simulink model "soc_WLAN_fpga"  (R2024b)
settings: Solver=FixedStepDiscrete  StartTime=0.0  StopTime=stopTime  RelTol=1e-3
PreLoadFcn:
  | addpath(fullfile(matlabroot,'toolbox','whdl','whdlexamples','whdlexamples'));
InitFcn:
  | addpath(fullfile(matlabroot,'toolbox','whdl','whdlexamples','whdlexamples'));
model workspace (MAT data in the model file):
  socvcb : containers.Map (value not decoded)
undefined symbols (not defined in the file): Add, bitRatePerOfdmSym, chanBW, coe, cpLen, dataUpsampleFactor, DelayValMaxNsdMinusLastPilotSc, DescramblerInitialSeed, designMultirateFIR, fftLen, filterLatency, filterUpsampleFactor, Fs, Hd, HT_MFMCS0, HT_MFMCS1, HT_MFMCS2, HT_MFMCS3, HT_MFMCS4, HT_MFMCS5, HT_MFMCS6, HT_MFMCS7, HTUnUsedScInd, inputSamplingRate, interp_coeff, maxPilotRefCounterVale, maxPilotsRef, maxPilotsRefNonHT, Ncol_HT, Ncol_NonHT, noDataSubCarriers, Non_HTMCS0, Non_HTMCS1, Non_HTMCS2, Non_HTMCS3, Non_HTMCS4, Non_HTMCS5, Non_HTMCS6, Non_HTMCS7, Nrow_HT, Nrow_NonHT, numDSC_HT, numDSC_HT_vhtSigB, numDSC_NonHT, numDscHT, numDscNonHT, numOfBitsPerOFDMSym, numOfDataBitsPerOFDMSym, numPilots, numScHT, numSCS_HT, numSCS_NonHT, pnSeq, QAM, rxDownsampleFactor, secondPIdx_HT, secondPIdx_NonHT, Shift, VHTMCS0, VHTMCS1 ... (+7)
libraries: hdlsllib x267, simulink x210, dspsigops x22, whdlutilities x10, whdlmod x9, dsphdlfiltering2 x5, dsphdlmathfun2 x4, whdledac x3, hwlogicconnlib x2, commhdlcrc x2, dsphdlsigops2 x2
(part 10 of 14)

== system soc_WLAN_fpga/WLAN/WLAN HDL/WLAN_Tx_Rx/WLAN_Rx/WLANHDLReceiver/DataRecovery/Deinterleaver/DeInterleaver_HT/Stage 2 64QAM/Write Logic/Handle Input Control Signals ==
  start : Inport
  valid : Inport  Port=2
  end : Inport  Port=3
  Delay{1..5} (5 alike) : Delay  DelayLength=1
  Generate Current Frame Status : Subsystem
  Generate Forced End : Subsystem
  Logical Operator : Logic  Operator=OR  IconShape=distinctive  AllPortsSameDT=off  OutDataTypeStr=boolean
  Logical Operator1 : Logic  Operator=NOT  IconShape=distinctive  AllPortsSameDT=off  OutDataTypeStr=boolean
  Logical Operator2 : Logic  IconShape=distinctive  AllPortsSameDT=off  OutDataTypeStr=boolean
  Logical Operator3 : Logic  Inputs=4  IconShape=distinctive  AllPortsSameDT=off  OutDataTypeStr=boolean
  Logical Operator5 : Logic  IconShape=distinctive  AllPortsSameDT=off  OutDataTypeStr=boolean
  reset : Outport
  countEnb : Outport  Port=2
  endOut : Outport  Port=3
  endReady : Outport  Port=4
  wires:
  Logical Operator1/1 -> Logical Operator3/4
  Logical Operator/1 -> Delay1/1, endReady/1
  Delay1/1 -> Generate Current Frame Status/2(end), Delay5/1, Logical Operator1/1
  Generate Forced End/1(forcedEnd) -> Logical Operator/2
  Logical Operator3/1 -> Logical Operator/1
  valid/1 -> Logical Operator3/1, Logical Operator2/2, Generate Forced End/2(valid), Delay4/1
  Delay5/1 -> endOut/1
  Delay3/1 -> countEnb/1
  Delay2/1 -> reset/1
  start/1 -> Logical Operator2/1
  Delay4/1 -> Logical Operator5/1
  end/1 -> Logical Operator3/2
  Logical Operator2/1 -> Generate Forced End/1(rst), Generate Current Frame Status/1(start), Delay2/1
  Generate Current Frame Status/1(frameOn) -> Generate Forced End/3(frameOn), Logical Operator3/3, Logical Operator5/2
  Logical Operator5/1 -> Delay3/1

== system soc_WLAN_fpga/WLAN/WLAN HDL/WLAN_Tx_Rx/WLAN_Rx/WLANHDLReceiver/DataRecovery/Deinterleaver/DeInterleaver_HT/Stage 2 BPSK/Generate Ready/Generate Ready2 ==
  fifoCount : Inport
  pop : Inport  Port=2
  Compare To Constant1 : simulink/Logic and Bit Operations/Compare To Constant  relop===  const=0  OutDataTypeStr=boolean
  Compare To Constant4 : simulink/Logic and Bit Operations/Compare To Constant  relop===  const=1  OutDataTypeStr=boolean
  Logical Operator1 : Logic  Operator=OR  IconShape=distinctive  AllPortsSameDT=off  OutDataTypeStr=boolean
  Logical Operator14 : Logic  IconShape=distinctive  AllPortsSameDT=off  OutDataTypeStr=boolean
  ready2 : Outport
  wires:
  Compare To Constant1/1 -> Logical Operator1/1
  Logical Operator1/1 -> ready2/1
  Logical Operator14/1 -> Logical Operator1/2
  Compare To Constant4/1 -> Logical Operator14/1
  pop/1 -> Logical Operator14/2
  fifoCount/1 -> Compare To Constant4/1, Compare To Constant1/1

== system soc_WLAN_fpga/WLAN/WLAN HDL/WLAN_Tx_Rx/WLAN_Rx/WLANHDLReceiver/DataRecovery/Deinterleaver/DeInterleaver_HT/Stage 2 BPSK/Read Logic/Generate Base Read Address ==
  readStart : Inport
  Constant1 : Constant  Value=0  OutDataTypeStr=fixdt(0,nextpow2(maxBlkSize+1),0)  SampleTime=-1
  Constant5 : Constant  Value=maxBlkSize  OutDataTypeStr=fixdt(0,nextpow2(maxBlkSize+1),0)  SampleTime=-1
  Logical Operator7 : Logic  Operator=NOT  IconShape=distinctive  AllPortsSameDT=off  OutDataTypeStr=boolean
  Switch1 : Switch  Criteria=u2 ~= 0  SaturateOnIntegerOverflow=off  InputSameDT=off
  Unit Delay Enabled Synchronous2 : hdlsllib/Discrete/Unit Delay Enabled Synchronous  InitialCondition=1  SampleTime=-1
  baseAddr : Outport
  wires:
  readStart/1 -> Unit Delay Enabled Synchronous2/2
  Logical Operator7/1 -> Unit Delay Enabled Synchronous2/1
  Switch1/1 -> baseAddr/1
  Constant5/1 -> Switch1/1
  Constant1/1 -> Switch1/3
  Unit Delay Enabled Synchronous2/1 -> Logical Operator7/1, Switch1/2

== system soc_WLAN_fpga/WLAN/WLAN HDL/WLAN_Tx_Rx/WLAN_Rx/WLANHDLReceiver/DataRecovery/Deinterleaver/DeInterleaver_HT/Stage 2 BPSK/Read Logic/Generate Output Control Signals ==
  blockLen : Inport
  blockValid : Inport  Port=2
  blockCount : Inport  Port=3
  Add : Sum  Inputs=+-
  Add1 : Sum  Inputs=+-
  Compare To Constant : simulink/Logic and Bit Operations/Compare To Constant  relop===  const=0  OutDataTypeStr=boolean
  Constant : Constant  Value=8  OutDataTypeStr=fixdt(0,nextpow2(8+1),0)  SampleTime=-1
  Constant1 : Constant  Value=false  SampleTime=-1
  Constant2 : Constant  Value=11  OutDataTypeStr=fixdt(0,nextpow2(11+1),0)  SampleTime=-1
  Constant3 : Constant  Value=false  SampleTime=-1
  Delay{,1,5..6,8} (5 alike) : Delay  DelayLength=1
  Logical Operator1 : Logic  IconShape=distinctive  AllPortsSameDT=off  OutDataTypeStr=boolean
  Logical Operator2 : Logic  IconShape=distinctive  AllPortsSameDT=off  OutDataTypeStr=boolean
  Logical Operator3 : Logic  Operator=NOR  IconShape=distinctive  AllPortsSameDT=off  OutDataTypeStr=boolean
  Logical Operator4 : Logic  Operator=OR  IconShape=distinctive  AllPortsSameDT=off  OutDataTypeStr=boolean
  Logical Operator8 : Logic  IconShape=distinctive  AllPortsSameDT=off  OutDataTypeStr=boolean
  Relational Operator : RelationalOperator  Operator===  OutDataTypeStr=boolean  InputSameDT=off
  Relational Operator1 : RelationalOperator  OutDataTypeStr=boolean  InputSameDT=off
  Relational Operator2 : RelationalOperator  Operator=<=  OutDataTypeStr=boolean  InputSameDT=off
  Relational Operator3 : RelationalOperator  OutDataTypeStr=boolean  InputSameDT=off
  Unit Delay Enabled Synchronous : hdlsllib/Discrete/Unit Delay Enabled Synchronous  InitialCondition=1  SampleTime=-1
  Unit Delay Enabled Synchronous1 : hdlsllib/Discrete/Unit Delay Enabled Synchronous  InitialCondition=1  SampleTime=-1
  start : Outport
  end : Outport  Port=2
  valid : Outport  Port=3
  pop : Outport  Port=4
  advPop : Outport  Port=5
  wires:
  blockLen/1 -> Relational Operator/2, Add/1, Add1/1, Relational Operator2/2
  Delay/1 -> start/1, Unit Delay Enabled Synchronous/2, Unit Delay Enabled Synchronous1/2
  blockCount/1 -> Compare To Constant/1, Relational Operator/1, Relational Operator2/1, Relational Operator1/1, Relational Operator3/1
  Unit Delay Enabled Synchronous1/1 -> Logical Operator3/2
  Relational Operator3/1 -> Delay1/1
  Add1/1 -> Relational Operator3/2
  Constant2/1 -> Add1/2
  Constant3/1 -> Unit Delay Enabled Synchronous1/1
  Delay1/1 -> Logical Operator3/1
  Logical Operator3/1 -> advPop/1
  Unit Delay Enabled Synchronous/1 -> Logical Operator4/2
  Delay8/1 -> Logical Operator4/1
  Logical Operator4/1 -> pop/1
  Delay6/1 -> valid/1
  Delay5/1 -> end/1
  Constant1/1 -> Unit Delay Enabled Synchronous/1
  Compare To Constant/1 -> Logical Operator8/2
  Relational Operator1/1 -> Delay8/1
  Add/1 -> Relational Operator1/2
  Constant/1 -> Add/2
  Relational Operator2/1 -> Logical Operator1/2
  Relational Operator/1 -> Logical Operator2/2
  blockValid/1 -> Logical Operator8/1, Logical Operator2/1, Logical Operator1/1
  Logical Operator2/1 -> Delay5/1
  Logical Operator8/1 -> Delay/1
  Logical Operator1/1 -> Delay6/1

== system soc_WLAN_fpga/WLAN/WLAN HDL/WLAN_Tx_Rx/WLAN_Rx/WLANHDLReceiver/DataRecovery/Deinterleaver/DeInterleaver_HT/Stage 2 BPSK/Read Logic/Generate Read Address ==
  note: 1) Add Subsystem or Model blocks as valid variant choices.
      | 2) You cannot connect blocks at this level. At simulation, connectivity is automatically
      | determined, based on the active variant and port name matching.
  blockLen : Inport
  enable : Inport  Port=2
  reset : Inport  Port=3
  Read Address of Deinterleaver : Subsystem  VariantControl=isInterleaver==0
  Read Address of Interleaver : Subsystem  VariantControl=isInterleaver==1
  blockDataCount : Outport
  currentAddr : Outport  Port=2

== system soc_WLAN_fpga/WLAN/WLAN HDL/WLAN_Tx_Rx/WLAN_Rx/WLANHDLReceiver/DataRecovery/Deinterleaver/DeInterleaver_HT/Stage 2 BPSK/Write Logic/Generate Write Address ==
  rst : Inport
  enb : Inport  Port=2
  end : Inport  Port=3
  Add : Sum  OutDataTypeStr=Inherit: Inherit via back propagation
  Constant : Constant  Value=0  OutDataTypeStr=fixdt(0,nextpow2(maxBlkSize+1),0)  SampleTime=-1
  Constant4 : Constant  Value=maxBlkSize  OutDataTypeStr=fixdt(0,nextpow2(maxBlkSize+1),0)  SampleTime=-1
  HDL Counter : hdlsllib/Sources/HDL Counter  CountType=Count limited  CountInit=0  CountStep=1  CountMax=maxBlkSize  CountFromType=Initial value  CountFrom=0  CountResetPort=on  CountLoadPort=off  CountEnbPort=on  CountDirPort=off  CountHitOutputPort=off  CountDataType=Unsigned  CountWordLen=nextpow2(maxBlkSize+1)  CountFracLen=0  CountSampTime=1
  Logical Operator7 : Logic  Operator=NOT  IconShape=distinctive  AllPortsSameDT=off  OutDataTypeStr=boolean
  Switch : Switch  Criteria=u2 ~= 0  SaturateOnIntegerOverflow=off  InputSameDT=off
  Unit Delay Enabled Synchronous2 : hdlsllib/Discrete/Unit Delay Enabled Synchronous  InitialCondition=0  SampleTime=-1
  wrAddr : Outport
  count : Outport  Port=2
  wires:
  Logical Operator7/1 -> Unit Delay Enabled Synchronous2/1
  end/1 -> Unit Delay Enabled Synchronous2/2
  Unit Delay Enabled Synchronous2/1 -> Switch/2, Logical Operator7/1
  Add/1 -> wrAddr/1
  HDL Counter/1 -> count/1, Add/1  "currentAddr"
  rst/1 -> HDL Counter/1
  Constant/1 -> Switch/3
  Constant4/1 -> Switch/1
  enb/1 -> HDL Counter/2
  Switch/1 -> Add/2  "baseAddr"

== system soc_WLAN_fpga/WLAN/WLAN HDL/WLAN_Tx_Rx/WLAN_Rx/WLANHDLReceiver/DataRecovery/Deinterleaver/DeInterleaver_HT/Stage 2 BPSK/Write Logic/Handle Input Control Signals ==
  start : Inport
  valid : Inport  Port=2
  end : Inport  Port=3
  Delay{1..5} (5 alike) : Delay  DelayLength=1
  Generate Current Frame Status : Subsystem
  Generate Forced End : Subsystem
  Logical Operator : Logic  Operator=OR  IconShape=distinctive  AllPortsSameDT=off  OutDataTypeStr=boolean
  Logical Operator1 : Logic  Operator=NOT  IconShape=distinctive  AllPortsSameDT=off  OutDataTypeStr=boolean
  Logical Operator2 : Logic  IconShape=distinctive  AllPortsSameDT=off  OutDataTypeStr=boolean
  Logical Operator3 : Logic  Inputs=4  IconShape=distinctive  AllPortsSameDT=off  OutDataTypeStr=boolean
  Logical Operator5 : Logic  IconShape=distinctive  AllPortsSameDT=off  OutDataTypeStr=boolean
  reset : Outport
  countEnb : Outport  Port=2
  endOut : Outport  Port=3
  endReady : Outport  Port=4
  wires:
  Logical Operator1/1 -> Logical Operator3/4
  Logical Operator/1 -> Delay1/1, endReady/1
  Delay1/1 -> Generate Current Frame Status/2(end), Delay5/1, Logical Operator1/1
  Generate Forced End/1(forcedEnd) -> Logical Operator/2
  Logical Operator3/1 -> Logical Operator/1
  valid/1 -> Logical Operator3/1, Logical Operator2/2, Generate Forced End/2(valid), Delay4/1
  Delay5/1 -> endOut/1
  Delay3/1 -> countEnb/1
  Delay2/1 -> reset/1
  start/1 -> Logical Operator2/1
  Delay4/1 -> Logical Operator5/1
  end/1 -> Logical Operator3/2
  Logical Operator2/1 -> Generate Forced End/1(rst), Generate Current Frame Status/1(start), Delay2/1
  Generate Current Frame Status/1(frameOn) -> Generate Forced End/3(frameOn), Logical Operator3/3, Logical Operator5/2
  Logical Operator5/1 -> Delay3/1

== system soc_WLAN_fpga/WLAN/WLAN HDL/WLAN_Tx_Rx/WLAN_Rx/WLANHDLReceiver/DataRecovery/Deinterleaver/DeInterleaver_HT/Stage 2 QPSK/Generate Ready/Generate Ready2 ==
  fifoCount : Inport
  pop : Inport  Port=2
  Compare To Constant1 : simulink/Logic and Bit Operations/Compare To Constant  relop===  const=0  OutDataTypeStr=boolean
  Compare To Constant4 : simulink/Logic and Bit Operations/Compare To Constant  relop===  const=1  OutDataTypeStr=boolean
  Logical Operator1 : Logic  Operator=OR  IconShape=distinctive  AllPortsSameDT=off  OutDataTypeStr=boolean
  Logical Operator14 : Logic  IconShape=distinctive  AllPortsSameDT=off  OutDataTypeStr=boolean
  ready2 : Outport
  wires:
  Compare To Constant1/1 -> Logical Operator1/1
  Logical Operator1/1 -> ready2/1
  Logical Operator14/1 -> Logical Operator1/2
  Compare To Constant4/1 -> Logical Operator14/1
  pop/1 -> Logical Operator14/2
  fifoCount/1 -> Compare To Constant4/1, Compare To Constant1/1

== system soc_WLAN_fpga/WLAN/WLAN HDL/WLAN_Tx_Rx/WLAN_Rx/WLANHDLReceiver/DataRecovery/Deinterleaver/DeInterleaver_HT/Stage 2 QPSK/Read Logic/Generate Base Read Address ==
  readStart : Inport
  Constant1 : Constant  Value=0  OutDataTypeStr=fixdt(0,nextpow2(maxBlkSize+1),0)  SampleTime=-1
  Constant5 : Constant  Value=maxBlkSize  OutDataTypeStr=fixdt(0,nextpow2(maxBlkSize+1),0)  SampleTime=-1
  Logical Operator7 : Logic  Operator=NOT  IconShape=distinctive  AllPortsSameDT=off  OutDataTypeStr=boolean
  Switch1 : Switch  Criteria=u2 ~= 0  SaturateOnIntegerOverflow=off  InputSameDT=off
  Unit Delay Enabled Synchronous2 : hdlsllib/Discrete/Unit Delay Enabled Synchronous  InitialCondition=1  SampleTime=-1
  baseAddr : Outport
  wires:
  readStart/1 -> Unit Delay Enabled Synchronous2/2
  Logical Operator7/1 -> Unit Delay Enabled Synchronous2/1
  Switch1/1 -> baseAddr/1
  Constant5/1 -> Switch1/1
  Constant1/1 -> Switch1/3
  Unit Delay Enabled Synchronous2/1 -> Logical Operator7/1, Switch1/2

== system soc_WLAN_fpga/WLAN/WLAN HDL/WLAN_Tx_Rx/WLAN_Rx/WLANHDLReceiver/DataRecovery/Deinterleaver/DeInterleaver_HT/Stage 2 QPSK/Read Logic/Generate Output Control Signals ==
  blockLen : Inport
  blockValid : Inport  Port=2
  blockCount : Inport  Port=3
  Add : Sum  Inputs=+-
  Add1 : Sum  Inputs=+-
  Compare To Constant : simulink/Logic and Bit Operations/Compare To Constant  relop===  const=0  OutDataTypeStr=boolean
  Constant : Constant  Value=8  OutDataTypeStr=fixdt(0,nextpow2(8+1),0)  SampleTime=-1
  Constant1 : Constant  Value=false  SampleTime=-1
  Constant2 : Constant  Value=11  OutDataTypeStr=fixdt(0,nextpow2(11+1),0)  SampleTime=-1
  Constant3 : Constant  Value=false  SampleTime=-1
  Delay{,1,5..6,8} (5 alike) : Delay  DelayLength=1
  Logical Operator1 : Logic  IconShape=distinctive  AllPortsSameDT=off  OutDataTypeStr=boolean
  Logical Operator2 : Logic  IconShape=distinctive  AllPortsSameDT=off  OutDataTypeStr=boolean
  Logical Operator3 : Logic  Operator=NOR  IconShape=distinctive  AllPortsSameDT=off  OutDataTypeStr=boolean
  Logical Operator4 : Logic  Operator=OR  IconShape=distinctive  AllPortsSameDT=off  OutDataTypeStr=boolean
  Logical Operator8 : Logic  IconShape=distinctive  AllPortsSameDT=off  OutDataTypeStr=boolean
  Relational Operator : RelationalOperator  Operator===  OutDataTypeStr=boolean  InputSameDT=off
  Relational Operator1 : RelationalOperator  OutDataTypeStr=boolean  InputSameDT=off
  Relational Operator2 : RelationalOperator  Operator=<=  OutDataTypeStr=boolean  InputSameDT=off
  Relational Operator3 : RelationalOperator  OutDataTypeStr=boolean  InputSameDT=off
  Unit Delay Enabled Synchronous : hdlsllib/Discrete/Unit Delay Enabled Synchronous  InitialCondition=1  SampleTime=-1
  Unit Delay Enabled Synchronous1 : hdlsllib/Discrete/Unit Delay Enabled Synchronous  InitialCondition=1  SampleTime=-1
  start : Outport
  end : Outport  Port=2
  valid : Outport  Port=3
  pop : Outport  Port=4
  advPop : Outport  Port=5
  wires:
  blockLen/1 -> Relational Operator/2, Add/1, Add1/1, Relational Operator2/2
  Delay/1 -> start/1, Unit Delay Enabled Synchronous/2, Unit Delay Enabled Synchronous1/2
  blockCount/1 -> Compare To Constant/1, Relational Operator/1, Relational Operator2/1, Relational Operator1/1, Relational Operator3/1
  Unit Delay Enabled Synchronous1/1 -> Logical Operator3/2
  Relational Operator3/1 -> Delay1/1
  Add1/1 -> Relational Operator3/2
  Constant2/1 -> Add1/2
  Constant3/1 -> Unit Delay Enabled Synchronous1/1
  Delay1/1 -> Logical Operator3/1
  Logical Operator3/1 -> advPop/1
  Unit Delay Enabled Synchronous/1 -> Logical Operator4/2
  Delay8/1 -> Logical Operator4/1
  Logical Operator4/1 -> pop/1
  Delay6/1 -> valid/1
  Delay5/1 -> end/1
  Constant1/1 -> Unit Delay Enabled Synchronous/1
  Compare To Constant/1 -> Logical Operator8/2
  Relational Operator1/1 -> Delay8/1
  Add/1 -> Relational Operator1/2
  Constant/1 -> Add/2
  Relational Operator2/1 -> Logical Operator1/2
  Relational Operator/1 -> Logical Operator2/2
  blockValid/1 -> Logical Operator8/1, Logical Operator2/1, Logical Operator1/1
  Logical Operator2/1 -> Delay5/1
  Logical Operator8/1 -> Delay/1
  Logical Operator1/1 -> Delay6/1

== system soc_WLAN_fpga/WLAN/WLAN HDL/WLAN_Tx_Rx/WLAN_Rx/WLANHDLReceiver/DataRecovery/Deinterleaver/DeInterleaver_HT/Stage 2 QPSK/Read Logic/Generate Read Address ==
  note: 1) Add Subsystem or Model blocks as valid variant choices.
      | 2) You cannot connect blocks at this level. At simulation, connectivity is automatically
      | determined, based on the active variant and port name matching.
  blockLen : Inport
  enable : Inport  Port=2
  reset : Inport  Port=3
  Read Address of Deinterleaver : Subsystem  VariantControl=isInterleaver==0
  Read Address of Interleaver : Subsystem  VariantControl=isInterleaver==1
  blockDataCount : Outport
  currentAddr : Outport  Port=2

== system soc_WLAN_fpga/WLAN/WLAN HDL/WLAN_Tx_Rx/WLAN_Rx/WLANHDLReceiver/DataRecovery/Deinterleaver/DeInterleaver_HT/Stage 2 QPSK/Write Logic/Generate Write Address ==
  rst : Inport
  enb : Inport  Port=2
  end : Inport  Port=3
  Add : Sum  OutDataTypeStr=Inherit: Inherit via back propagation
  Constant : Constant  Value=0  OutDataTypeStr=fixdt(0,nextpow2(maxBlkSize+1),0)  SampleTime=-1
  Constant4 : Constant  Value=maxBlkSize  OutDataTypeStr=fixdt(0,nextpow2(maxBlkSize+1),0)  SampleTime=-1
  HDL Counter : hdlsllib/Sources/HDL Counter  CountType=Count limited  CountInit=0  CountStep=1  CountMax=maxBlkSize  CountFromType=Initial value  CountFrom=0  CountResetPort=on  CountLoadPort=off  CountEnbPort=on  CountDirPort=off  CountHitOutputPort=off  CountDataType=Unsigned  CountWordLen=nextpow2(maxBlkSize+1)  CountFracLen=0  CountSampTime=1
  Logical Operator7 : Logic  Operator=NOT  IconShape=distinctive  AllPortsSameDT=off  OutDataTypeStr=boolean
  Switch : Switch  Criteria=u2 ~= 0  SaturateOnIntegerOverflow=off  InputSameDT=off
  Unit Delay Enabled Synchronous2 : hdlsllib/Discrete/Unit Delay Enabled Synchronous  InitialCondition=0  SampleTime=-1
  wrAddr : Outport
  count : Outport  Port=2
  wires:
  Logical Operator7/1 -> Unit Delay Enabled Synchronous2/1
  end/1 -> Unit Delay Enabled Synchronous2/2
  Unit Delay Enabled Synchronous2/1 -> Switch/2, Logical Operator7/1
  Add/1 -> wrAddr/1
  HDL Counter/1 -> count/1, Add/1  "currentAddr"
  rst/1 -> HDL Counter/1
  Constant/1 -> Switch/3
  Constant4/1 -> Switch/1
  enb/1 -> HDL Counter/2
  Switch/1 -> Add/2  "baseAddr"

== system soc_WLAN_fpga/WLAN/WLAN HDL/WLAN_Tx_Rx/WLAN_Rx/WLANHDLReceiver/DataRecovery/Deinterleaver/DeInterleaver_HT/Stage 2 QPSK/Write Logic/Handle Input Control Signals ==
  start : Inport
  valid : Inport  Port=2
  end : Inport  Port=3
  Delay{1..5} (5 alike) : Delay  DelayLength=1
  Generate Current Frame Status : Subsystem
  Generate Forced End : Subsystem
  Logical Operator : Logic  Operator=OR  IconShape=distinctive  AllPortsSameDT=off  OutDataTypeStr=boolean
  Logical Operator1 : Logic  Operator=NOT  IconShape=distinctive  AllPortsSameDT=off  OutDataTypeStr=boolean
  Logical Operator2 : Logic  IconShape=distinctive  AllPortsSameDT=off  OutDataTypeStr=boolean
  Logical Operator3 : Logic  Inputs=4  IconShape=distinctive  AllPortsSameDT=off  OutDataTypeStr=boolean
  Logical Operator5 : Logic  IconShape=distinctive  AllPortsSameDT=off  OutDataTypeStr=boolean
  reset : Outport
  countEnb : Outport  Port=2
  endOut : Outport  Port=3
  endReady : Outport  Port=4
  wires:
  Logical Operator1/1 -> Logical Operator3/4
  Logical Operator/1 -> Delay1/1, endReady/1
  Delay1/1 -> Generate Current Frame Status/2(end), Delay5/1, Logical Operator1/1
  Generate Forced End/1(forcedEnd) -> Logical Operator/2
  Logical Operator3/1 -> Logical Operator/1
  valid/1 -> Logical Operator3/1, Logical Operator2/2, Generate Forced End/2(valid), Delay4/1
  Delay5/1 -> endOut/1
  Delay3/1 -> countEnb/1
  Delay2/1 -> reset/1
  start/1 -> Logical Operator2/1
  Delay4/1 -> Logical Operator5/1
  end/1 -> Logical Operator3/2
  Logical Operator2/1 -> Generate Forced End/1(rst), Generate Current Frame Status/1(start), Delay2/1
  Generate Current Frame Status/1(frameOn) -> Generate Forced End/3(frameOn), Logical Operator3/3, Logical Operator5/2
  Logical Operator5/1 -> Delay3/1

== system soc_WLAN_fpga/WLAN/WLAN HDL/WLAN_Tx_Rx/WLAN_Rx/WLANHDLReceiver/DataRecovery/Deinterleaver/DeInterleaver_NonHT/Stage 2 16QAM /Generate Ready/Generate Ready2 ==
  fifoCount : Inport
  pop : Inport  Port=2
  Compare To Constant1 : simulink/Logic and Bit Operations/Compare To Constant  relop===  const=0  OutDataTypeStr=boolean
  Compare To Constant4 : simulink/Logic and Bit Operations/Compare To Constant  relop===  const=1  OutDataTypeStr=boolean
  Logical Operator1 : Logic  Operator=OR  IconShape=distinctive  AllPortsSameDT=off  OutDataTypeStr=boolean
  Logical Operator14 : Logic  IconShape=distinctive  AllPortsSameDT=off  OutDataTypeStr=boolean
  ready2 : Outport
  wires:
  Compare To Constant1/1 -> Logical Operator1/1
  Logical Operator1/1 -> ready2/1
  Logical Operator14/1 -> Logical Operator1/2
  Compare To Constant4/1 -> Logical Operator14/1
  pop/1 -> Logical Operator14/2
  fifoCount/1 -> Compare To Constant4/1, Compare To Constant1/1

== system soc_WLAN_fpga/WLAN/WLAN HDL/WLAN_Tx_Rx/WLAN_Rx/WLANHDLReceiver/DataRecovery/Deinterleaver/DeInterleaver_NonHT/Stage 2 16QAM /Read Logic/Generate Base Read Address ==
  readStart : Inport
  Constant1 : Constant  Value=0  OutDataTypeStr=fixdt(0,nextpow2(maxBlkSize+1),0)  SampleTime=-1
  Constant5 : Constant  Value=maxBlkSize  OutDataTypeStr=fixdt(0,nextpow2(maxBlkSize+1),0)  SampleTime=-1
  Logical Operator7 : Logic  Operator=NOT  IconShape=distinctive  AllPortsSameDT=off  OutDataTypeStr=boolean
  Switch1 : Switch  Criteria=u2 ~= 0  SaturateOnIntegerOverflow=off  InputSameDT=off
  Unit Delay Enabled Synchronous2 : hdlsllib/Discrete/Unit Delay Enabled Synchronous  InitialCondition=1  SampleTime=-1
  baseAddr : Outport
  wires:
  readStart/1 -> Unit Delay Enabled Synchronous2/2
  Logical Operator7/1 -> Unit Delay Enabled Synchronous2/1
  Switch1/1 -> baseAddr/1
  Constant5/1 -> Switch1/1
  Constant1/1 -> Switch1/3
  Unit Delay Enabled Synchronous2/1 -> Logical Operator7/1, Switch1/2

== system soc_WLAN_fpga/WLAN/WLAN HDL/WLAN_Tx_Rx/WLAN_Rx/WLANHDLReceiver/DataRecovery/Deinterleaver/DeInterleaver_NonHT/Stage 2 16QAM /Read Logic/Generate Output Control Signals ==
  blockLen : Inport
  blockValid : Inport  Port=2
  blockCount : Inport  Port=3
  Add : Sum  Inputs=+-
  Add1 : Sum  Inputs=+-
  Compare To Constant : simulink/Logic and Bit Operations/Compare To Constant  relop===  const=0  OutDataTypeStr=boolean
  Constant : Constant  Value=8  OutDataTypeStr=fixdt(0,nextpow2(8+1),0)  SampleTime=-1
  Constant1 : Constant  Value=false  SampleTime=-1
  Constant2 : Constant  Value=11  OutDataTypeStr=fixdt(0,nextpow2(11+1),0)  SampleTime=-1
  Constant3 : Constant  Value=false  SampleTime=-1
  Delay{,1,5..6,8} (5 alike) : Delay  DelayLength=1
  Logical Operator1 : Logic  IconShape=distinctive  AllPortsSameDT=off  OutDataTypeStr=boolean
  Logical Operator2 : Logic  IconShape=distinctive  AllPortsSameDT=off  OutDataTypeStr=boolean
  Logical Operator3 : Logic  Operator=NOR  IconShape=distinctive  AllPortsSameDT=off  OutDataTypeStr=boolean
  Logical Operator4 : Logic  Operator=OR  IconShape=distinctive  AllPortsSameDT=off  OutDataTypeStr=boolean
  Logical Operator8 : Logic  IconShape=distinctive  AllPortsSameDT=off  OutDataTypeStr=boolean
  Relational Operator : RelationalOperator  Operator===  OutDataTypeStr=boolean  InputSameDT=off
  Relational Operator1 : RelationalOperator  OutDataTypeStr=boolean  InputSameDT=off
  Relational Operator2 : RelationalOperator  Operator=<=  OutDataTypeStr=boolean  InputSameDT=off
  Relational Operator3 : RelationalOperator  OutDataTypeStr=boolean  InputSameDT=off
  Unit Delay Enabled Synchronous : hdlsllib/Discrete/Unit Delay Enabled Synchronous  InitialCondition=1  SampleTime=-1
  Unit Delay Enabled Synchronous1 : hdlsllib/Discrete/Unit Delay Enabled Synchronous  InitialCondition=1  SampleTime=-1
  start : Outport
  end : Outport  Port=2
  valid : Outport  Port=3
  pop : Outport  Port=4
  advPop : Outport  Port=5
  wires:
  blockLen/1 -> Relational Operator/2, Add/1, Add1/1, Relational Operator2/2
  Delay/1 -> start/1, Unit Delay Enabled Synchronous/2, Unit Delay Enabled Synchronous1/2
  blockCount/1 -> Compare To Constant/1, Relational Operator/1, Relational Operator2/1, Relational Operator1/1, Relational Operator3/1
  Unit Delay Enabled Synchronous1/1 -> Logical Operator3/2
  Relational Operator3/1 -> Delay1/1
  Add1/1 -> Relational Operator3/2
  Constant2/1 -> Add1/2
  Constant3/1 -> Unit Delay Enabled Synchronous1/1
  Delay1/1 -> Logical Operator3/1
  Logical Operator3/1 -> advPop/1
  Unit Delay Enabled Synchronous/1 -> Logical Operator4/2
  Delay8/1 -> Logical Operator4/1
  Logical Operator4/1 -> pop/1
  Delay6/1 -> valid/1
  Delay5/1 -> end/1
  Constant1/1 -> Unit Delay Enabled Synchronous/1
  Compare To Constant/1 -> Logical Operator8/2
  Relational Operator1/1 -> Delay8/1
  Add/1 -> Relational Operator1/2
  Constant/1 -> Add/2
  Relational Operator2/1 -> Logical Operator1/2
  Relational Operator/1 -> Logical Operator2/2
  blockValid/1 -> Logical Operator8/1, Logical Operator2/1, Logical Operator1/1
  Logical Operator2/1 -> Delay5/1
  Logical Operator8/1 -> Delay/1
  Logical Operator1/1 -> Delay6/1

== system soc_WLAN_fpga/WLAN/WLAN HDL/WLAN_Tx_Rx/WLAN_Rx/WLANHDLReceiver/DataRecovery/Deinterleaver/DeInterleaver_NonHT/Stage 2 16QAM /Read Logic/Generate Read Address ==
  note: 1) Add Subsystem or Model blocks as valid variant choices.
      | 2) You cannot connect blocks at this level. At simulation, connectivity is automatically
      | determined, based on the active variant and port name matching.
  blockLen : Inport
  enable : Inport  Port=2
  reset : Inport  Port=3
  Read Address of Deinterleaver : Subsystem  VariantControl=isInterleaver==0
  Read Address of Interleaver : Subsystem  VariantControl=isInterleaver==1
  blockDataCount : Outport
  currentAddr : Outport  Port=2

== system soc_WLAN_fpga/WLAN/WLAN HDL/WLAN_Tx_Rx/WLAN_Rx/WLANHDLReceiver/DataRecovery/Deinterleaver/DeInterleaver_NonHT/Stage 2 16QAM /Write Logic/Generate Write Address ==
  rst : Inport
  enb : Inport  Port=2
  end : Inport  Port=3
  Add : Sum  OutDataTypeStr=Inherit: Inherit via back propagation
  Constant : Constant  Value=0  OutDataTypeStr=fixdt(0,nextpow2(maxBlkSize+1),0)  SampleTime=-1
  Constant4 : Constant  Value=maxBlkSize  OutDataTypeStr=fixdt(0,nextpow2(maxBlkSize+1),0)  SampleTime=-1
  HDL Counter : hdlsllib/Sources/HDL Counter  CountType=Count limited  CountInit=0  CountStep=1  CountMax=maxBlkSize  CountFromType=Initial value  CountFrom=0  CountResetPort=on  CountLoadPort=off  CountEnbPort=on  CountDirPort=off  CountHitOutputPort=off  CountDataType=Unsigned  CountWordLen=nextpow2(maxBlkSize+1)  CountFracLen=0  CountSampTime=1
  Logical Operator7 : Logic  Operator=NOT  IconShape=distinctive  AllPortsSameDT=off  OutDataTypeStr=boolean
  Switch : Switch  Criteria=u2 ~= 0  SaturateOnIntegerOverflow=off  InputSameDT=off
  Unit Delay Enabled Synchronous2 : hdlsllib/Discrete/Unit Delay Enabled Synchronous  InitialCondition=0  SampleTime=-1
  wrAddr : Outport
  count : Outport  Port=2
  wires:
  Logical Operator7/1 -> Unit Delay Enabled Synchronous2/1
  end/1 -> Unit Delay Enabled Synchronous2/2
  Unit Delay Enabled Synchronous2/1 -> Switch/2, Logical Operator7/1
  Add/1 -> wrAddr/1
  HDL Counter/1 -> count/1, Add/1  "currentAddr"
  rst/1 -> HDL Counter/1
  Constant/1 -> Switch/3
  Constant4/1 -> Switch/1
  enb/1 -> HDL Counter/2
  Switch/1 -> Add/2  "baseAddr"

== system soc_WLAN_fpga/WLAN/WLAN HDL/WLAN_Tx_Rx/WLAN_Rx/WLANHDLReceiver/DataRecovery/Deinterleaver/DeInterleaver_NonHT/Stage 2 16QAM /Write Logic/Handle Input Control Signals ==
  start : Inport
  valid : Inport  Port=2
  end : Inport  Port=3
  Delay{1..5} (5 alike) : Delay  DelayLength=1
  Generate Current Frame Status : Subsystem
  Generate Forced End : Subsystem
  Logical Operator : Logic  Operator=OR  IconShape=distinctive  AllPortsSameDT=off  OutDataTypeStr=boolean
  Logical Operator1 : Logic  Operator=NOT  IconShape=distinctive  AllPortsSameDT=off  OutDataTypeStr=boolean
  Logical Operator2 : Logic  IconShape=distinctive  AllPortsSameDT=off  OutDataTypeStr=boolean
  Logical Operator3 : Logic  Inputs=4  IconShape=distinctive  AllPortsSameDT=off  OutDataTypeStr=boolean
  Logical Operator5 : Logic  IconShape=distinctive  AllPortsSameDT=off  OutDataTypeStr=boolean
  reset : Outport
  countEnb : Outport  Port=2
  endOut : Outport  Port=3
  endReady : Outport  Port=4
  wires:
  Logical Operator1/1 -> Logical Operator3/4
  Logical Operator/1 -> Delay1/1, endReady/1
  Delay1/1 -> Generate Current Frame Status/2(end), Delay5/1, Logical Operator1/1
  Generate Forced End/1(forcedEnd) -> Logical Operator/2
  Logical Operator3/1 -> Logical Operator/1
  valid/1 -> Logical Operator3/1, Logical Operator2/2, Generate Forced End/2(valid), Delay4/1
  Delay5/1 -> endOut/1
  Delay3/1 -> countEnb/1
  Delay2/1 -> reset/1
  start/1 -> Logical Operator2/1
  Delay4/1 -> Logical Operator5/1
  end/1 -> Logical Operator3/2
  Logical Operator2/1 -> Generate Forced End/1(rst), Generate Current Frame Status/1(start), Delay2/1
  Generate Current Frame Status/1(frameOn) -> Generate Forced End/3(frameOn), Logical Operator3/3, Logical Operator5/2
  Logical Operator5/1 -> Delay3/1

== system soc_WLAN_fpga/WLAN/WLAN HDL/WLAN_Tx_Rx/WLAN_Rx/WLANHDLReceiver/DataRecovery/Deinterleaver/DeInterleaver_NonHT/Stage 2 64QAM/Generate Ready/Generate Ready2 ==
  fifoCount : Inport
  pop : Inport  Port=2
  Compare To Constant1 : simulink/Logic and Bit Operations/Compare To Constant  relop===  const=0  OutDataTypeStr=boolean
  Compare To Constant4 : simulink/Logic and Bit Operations/Compare To Constant  relop===  const=1  OutDataTypeStr=boolean
  Logical Operator1 : Logic  Operator=OR  IconShape=distinctive  AllPortsSameDT=off  OutDataTypeStr=boolean
  Logical Operator14 : Logic  IconShape=distinctive  AllPortsSameDT=off  OutDataTypeStr=boolean
  ready2 : Outport
  wires:
  Compare To Constant1/1 -> Logical Operator1/1
  Logical Operator1/1 -> ready2/1
  Logical Operator14/1 -> Logical Operator1/2
  Compare To Constant4/1 -> Logical Operator14/1
  pop/1 -> Logical Operator14/2
  fifoCount/1 -> Compare To Constant4/1, Compare To Constant1/1

== system soc_WLAN_fpga/WLAN/WLAN HDL/WLAN_Tx_Rx/WLAN_Rx/WLANHDLReceiver/DataRecovery/Deinterleaver/DeInterleaver_NonHT/Stage 2 64QAM/Read Logic/Generate Base Read Address ==
  readStart : Inport
  Constant1 : Constant  Value=0  OutDataTypeStr=fixdt(0,nextpow2(maxBlkSize+1),0)  SampleTime=-1
  Constant5 : Constant  Value=maxBlkSize  OutDataTypeStr=fixdt(0,nextpow2(maxBlkSize+1),0)  SampleTime=-1
  Logical Operator7 : Logic  Operator=NOT  IconShape=distinctive  AllPortsSameDT=off  OutDataTypeStr=boolean
  Switch1 : Switch  Criteria=u2 ~= 0  SaturateOnIntegerOverflow=off  InputSameDT=off
  Unit Delay Enabled Synchronous2 : hdlsllib/Discrete/Unit Delay Enabled Synchronous  InitialCondition=1  SampleTime=-1
  baseAddr : Outport
  wires:
  readStart/1 -> Unit Delay Enabled Synchronous2/2
  Logical Operator7/1 -> Unit Delay Enabled Synchronous2/1
  Switch1/1 -> baseAddr/1
  Constant5/1 -> Switch1/1
  Constant1/1 -> Switch1/3
  Unit Delay Enabled Synchronous2/1 -> Logical Operator7/1, Switch1/2

== system soc_WLAN_fpga/WLAN/WLAN HDL/WLAN_Tx_Rx/WLAN_Rx/WLANHDLReceiver/DataRecovery/Deinterleaver/DeInterleaver_NonHT/Stage 2 64QAM/Read Logic/Generate Output Control Signals ==
  blockLen : Inport
  blockValid : Inport  Port=2
  blockCount : Inport  Port=3
  Add : Sum  Inputs=+-
  Add1 : Sum  Inputs=+-
  Compare To Constant : simulink/Logic and Bit Operations/Compare To Constant  relop===  const=0  OutDataTypeStr=boolean
  Constant : Constant  Value=8  OutDataTypeStr=fixdt(0,nextpow2(8+1),0)  SampleTime=-1
  Constant1 : Constant  Value=false  SampleTime=-1
  Constant2 : Constant  Value=11  OutDataTypeStr=fixdt(0,nextpow2(11+1),0)  SampleTime=-1
  Constant3 : Constant  Value=false  SampleTime=-1
  Delay{,1,5..6,8} (5 alike) : Delay  DelayLength=1
  Logical Operator1 : Logic  IconShape=distinctive  AllPortsSameDT=off  OutDataTypeStr=boolean
  Logical Operator2 : Logic  IconShape=distinctive  AllPortsSameDT=off  OutDataTypeStr=boolean
  Logical Operator3 : Logic  Operator=NOR  IconShape=distinctive  AllPortsSameDT=off  OutDataTypeStr=boolean
  Logical Operator4 : Logic  Operator=OR  IconShape=distinctive  AllPortsSameDT=off  OutDataTypeStr=boolean
  Logical Operator8 : Logic  IconShape=distinctive  AllPortsSameDT=off  OutDataTypeStr=boolean
  Relational Operator : RelationalOperator  Operator===  OutDataTypeStr=boolean  InputSameDT=off
  Relational Operator1 : RelationalOperator  OutDataTypeStr=boolean  InputSameDT=off
  Relational Operator2 : RelationalOperator  Operator=<=  OutDataTypeStr=boolean  InputSameDT=off
  Relational Operator3 : RelationalOperator  OutDataTypeStr=boolean  InputSameDT=off
  Unit Delay Enabled Synchronous : hdlsllib/Discrete/Unit Delay Enabled Synchronous  InitialCondition=1  SampleTime=-1
  Unit Delay Enabled Synchronous1 : hdlsllib/Discrete/Unit Delay Enabled Synchronous  InitialCondition=1  SampleTime=-1
  start : Outport
  end : Outport  Port=2
  valid : Outport  Port=3
  pop : Outport  Port=4
  advPop : Outport  Port=5
  wires:
  blockLen/1 -> Relational Operator/2, Add/1, Add1/1, Relational Operator2/2
  Delay/1 -> start/1, Unit Delay Enabled Synchronous/2, Unit Delay Enabled Synchronous1/2
  blockCount/1 -> Compare To Constant/1, Relational Operator/1, Relational Operator2/1, Relational Operator1/1, Relational Operator3/1
  Unit Delay Enabled Synchronous1/1 -> Logical Operator3/2
  Relational Operator3/1 -> Delay1/1
  Add1/1 -> Relational Operator3/2
  Constant2/1 -> Add1/2
  Constant3/1 -> Unit Delay Enabled Synchronous1/1
  Delay1/1 -> Logical Operator3/1
  Logical Operator3/1 -> advPop/1
  Unit Delay Enabled Synchronous/1 -> Logical Operator4/2
  Delay8/1 -> Logical Operator4/1
  Logical Operator4/1 -> pop/1
  Delay6/1 -> valid/1
  Delay5/1 -> end/1
  Constant1/1 -> Unit Delay Enabled Synchronous/1
  Compare To Constant/1 -> Logical Operator8/2
  Relational Operator1/1 -> Delay8/1
  Add/1 -> Relational Operator1/2
  Constant/1 -> Add/2
  Relational Operator2/1 -> Logical Operator1/2
  Relational Operator/1 -> Logical Operator2/2
  blockValid/1 -> Logical Operator8/1, Logical Operator2/1, Logical Operator1/1
  Logical Operator2/1 -> Delay5/1
  Logical Operator8/1 -> Delay/1
  Logical Operator1/1 -> Delay6/1

== system soc_WLAN_fpga/WLAN/WLAN HDL/WLAN_Tx_Rx/WLAN_Rx/WLANHDLReceiver/DataRecovery/Deinterleaver/DeInterleaver_NonHT/Stage 2 64QAM/Read Logic/Generate Read Address ==
  note: 1) Add Subsystem or Model blocks as valid variant choices.
      | 2) You cannot connect blocks at this level. At simulation, connectivity is automatically
      | determined, based on the active variant and port name matching.
  blockLen : Inport
  enable : Inport  Port=2
  reset : Inport  Port=3
  Read Address of Deinterleaver : Subsystem  VariantControl=isInterleaver==0
  Read Address of Interleaver : Subsystem  VariantControl=isInterleaver==1
  blockDataCount : Outport
  currentAddr : Outport  Port=2

== system soc_WLAN_fpga/WLAN/WLAN HDL/WLAN_Tx_Rx/WLAN_Rx/WLANHDLReceiver/DataRecovery/Deinterleaver/DeInterleaver_NonHT/Stage 2 64QAM/Write Logic/Generate Write Address ==
  rst : Inport
  enb : Inport  Port=2
  end : Inport  Port=3
  Add : Sum  OutDataTypeStr=Inherit: Inherit via back propagation
  Constant : Constant  Value=0  OutDataTypeStr=fixdt(0,nextpow2(maxBlkSize+1),0)  SampleTime=-1
  Constant4 : Constant  Value=maxBlkSize  OutDataTypeStr=fixdt(0,nextpow2(maxBlkSize+1),0)  SampleTime=-1
  HDL Counter : hdlsllib/Sources/HDL Counter  CountType=Count limited  CountInit=0  CountStep=1  CountMax=maxBlkSize  CountFromType=Initial value  CountFrom=0  CountResetPort=on  CountLoadPort=off  CountEnbPort=on  CountDirPort=off  CountHitOutputPort=off  CountDataType=Unsigned  CountWordLen=nextpow2(maxBlkSize+1)  CountFracLen=0  CountSampTime=1
  Logical Operator7 : Logic  Operator=NOT  IconShape=distinctive  AllPortsSameDT=off  OutDataTypeStr=boolean
  Switch : Switch  Criteria=u2 ~= 0  SaturateOnIntegerOverflow=off  InputSameDT=off
  Unit Delay Enabled Synchronous2 : hdlsllib/Discrete/Unit Delay Enabled Synchronous  InitialCondition=0  SampleTime=-1
  wrAddr : Outport
  count : Outport  Port=2
  wires:
  Logical Operator7/1 -> Unit Delay Enabled Synchronous2/1
  end/1 -> Unit Delay Enabled Synchronous2/2
  Unit Delay Enabled Synchronous2/1 -> Switch/2, Logical Operator7/1
  Add/1 -> wrAddr/1
  HDL Counter/1 -> count/1, Add/1  "currentAddr"
  rst/1 -> HDL Counter/1
  Constant/1 -> Switch/3
  Constant4/1 -> Switch/1
  enb/1 -> HDL Counter/2
  Switch/1 -> Add/2  "baseAddr"

== system soc_WLAN_fpga/WLAN/WLAN HDL/WLAN_Tx_Rx/WLAN_Rx/WLANHDLReceiver/DataRecovery/Deinterleaver/DeInterleaver_NonHT/Stage 2 64QAM/Write Logic/Handle Input Control Signals ==
  start : Inport
  valid : Inport  Port=2
  end : Inport  Port=3
  Delay{1..5} (5 alike) : Delay  DelayLength=1
  Generate Current Frame Status : Subsystem
  Generate Forced End : Subsystem
  Logical Operator : Logic  Operator=OR  IconShape=distinctive  AllPortsSameDT=off  OutDataTypeStr=boolean
  Logical Operator1 : Logic  Operator=NOT  IconShape=distinctive  AllPortsSameDT=off  OutDataTypeStr=boolean
  Logical Operator2 : Logic  IconShape=distinctive  AllPortsSameDT=off  OutDataTypeStr=boolean
  Logical Operator3 : Logic  Inputs=4  IconShape=distinctive  AllPortsSameDT=off  OutDataTypeStr=boolean
  Logical Operator5 : Logic  IconShape=distinctive  AllPortsSameDT=off  OutDataTypeStr=boolean
  reset : Outport
  countEnb : Outport  Port=2
  endOut : Outport  Port=3
  endReady : Outport  Port=4
  wires:
  Logical Operator1/1 -> Logical Operator3/4
  Logical Operator/1 -> Delay1/1, endReady/1
  Delay1/1 -> Generate Current Frame Status/2(end), Delay5/1, Logical Operator1/1
  Generate Forced End/1(forcedEnd) -> Logical Operator/2
  Logical Operator3/1 -> Logical Operator/1
  valid/1 -> Logical Operator3/1, Logical Operator2/2, Generate Forced End/2(valid), Delay4/1
  Delay5/1 -> endOut/1
  Delay3/1 -> countEnb/1
  Delay2/1 -> reset/1
  start/1 -> Logical Operator2/1
  Delay4/1 -> Logical Operator5/1
  end/1 -> Logical Operator3/2
  Logical Operator2/1 -> Generate Forced End/1(rst), Generate Current Frame Status/1(start), Delay2/1
  Generate Current Frame Status/1(frameOn) -> Generate Forced End/3(frameOn), Logical Operator3/3, Logical Operator5/2
  Logical Operator5/1 -> Delay3/1

== system soc_WLAN_fpga/WLAN/WLAN HDL/WLAN_Tx_Rx/WLAN_Rx/WLANHDLReceiver/DataRecovery/Deinterleaver/DeInterleaver_NonHT/Stage 2 BPSK/Generate Ready/Generate Ready2 ==
  fifoCount : Inport
  pop : Inport  Port=2
  Compare To Constant1 : simulink/Logic and Bit Operations/Compare To Constant  relop===  const=0  OutDataTypeStr=boolean
  Compare To Constant4 : simulink/Logic and Bit Operations/Compare To Constant  relop===  const=1  OutDataTypeStr=boolean
  Logical Operator1 : Logic  Operator=OR  IconShape=distinctive  AllPortsSameDT=off  OutDataTypeStr=boolean
  Logical Operator14 : Logic  IconShape=distinctive  AllPortsSameDT=off  OutDataTypeStr=boolean
  ready2 : Outport
  wires:
  Compare To Constant1/1 -> Logical Operator1/1
  Logical Operator1/1 -> ready2/1
  Logical Operator14/1 -> Logical Operator1/2
  Compare To Constant4/1 -> Logical Operator14/1
  pop/1 -> Logical Operator14/2
  fifoCount/1 -> Compare To Constant4/1, Compare To Constant1/1

== system soc_WLAN_fpga/WLAN/WLAN HDL/WLAN_Tx_Rx/WLAN_Rx/WLANHDLReceiver/DataRecovery/Deinterleaver/DeInterleaver_NonHT/Stage 2 BPSK/Read Logic/Generate Base Read Address ==
  readStart : Inport
  Constant1 : Constant  Value=0  OutDataTypeStr=fixdt(0,nextpow2(maxBlkSize+1),0)  SampleTime=-1
  Constant5 : Constant  Value=maxBlkSize  OutDataTypeStr=fixdt(0,nextpow2(maxBlkSize+1),0)  SampleTime=-1
  Logical Operator7 : Logic  Operator=NOT  IconShape=distinctive  AllPortsSameDT=off  OutDataTypeStr=boolean
  Switch1 : Switch  Criteria=u2 ~= 0  SaturateOnIntegerOverflow=off  InputSameDT=off
  Unit Delay Enabled Synchronous2 : hdlsllib/Discrete/Unit Delay Enabled Synchronous  InitialCondition=1  SampleTime=-1
  baseAddr : Outport
  wires:
  readStart/1 -> Unit Delay Enabled Synchronous2/2
  Logical Operator7/1 -> Unit Delay Enabled Synchronous2/1
  Switch1/1 -> baseAddr/1
  Constant5/1 -> Switch1/1
  Constant1/1 -> Switch1/3
  Unit Delay Enabled Synchronous2/1 -> Logical Operator7/1, Switch1/2

== system soc_WLAN_fpga/WLAN/WLAN HDL/WLAN_Tx_Rx/WLAN_Rx/WLANHDLReceiver/DataRecovery/Deinterleaver/DeInterleaver_NonHT/Stage 2 BPSK/Read Logic/Generate Output Control Signals ==
  blockLen : Inport
  blockValid : Inport  Port=2
  blockCount : Inport  Port=3
  Add : Sum  Inputs=+-
  Add1 : Sum  Inputs=+-
  Compare To Constant : simulink/Logic and Bit Operations/Compare To Constant  relop===  const=0  OutDataTypeStr=boolean
  Constant : Constant  Value=8  OutDataTypeStr=fixdt(0,nextpow2(8+1),0)  SampleTime=-1
  Constant1 : Constant  Value=false  SampleTime=-1
  Constant2 : Constant  Value=11  OutDataTypeStr=fixdt(0,nextpow2(11+1),0)  SampleTime=-1
  Constant3 : Constant  Value=false  SampleTime=-1
  Delay{,1,5..6,8} (5 alike) : Delay  DelayLength=1
  Logical Operator1 : Logic  IconShape=distinctive  AllPortsSameDT=off  OutDataTypeStr=boolean
  Logical Operator2 : Logic  IconShape=distinctive  AllPortsSameDT=off  OutDataTypeStr=boolean
  Logical Operator3 : Logic  Operator=NOR  IconShape=distinctive  AllPortsSameDT=off  OutDataTypeStr=boolean
  Logical Operator4 : Logic  Operator=OR  IconShape=distinctive  AllPortsSameDT=off  OutDataTypeStr=boolean
  Logical Operator8 : Logic  IconShape=distinctive  AllPortsSameDT=off  OutDataTypeStr=boolean
  Relational Operator : RelationalOperator  Operator===  OutDataTypeStr=boolean  InputSameDT=off
  Relational Operator1 : RelationalOperator  OutDataTypeStr=boolean  InputSameDT=off
  Relational Operator2 : RelationalOperator  Operator=<=  OutDataTypeStr=boolean  InputSameDT=off
  Relational Operator3 : RelationalOperator  OutDataTypeStr=boolean  InputSameDT=off
  Unit Delay Enabled Synchronous : hdlsllib/Discrete/Unit Delay Enabled Synchronous  InitialCondition=1  SampleTime=-1
  Unit Delay Enabled Synchronous1 : hdlsllib/Discrete/Unit Delay Enabled Synchronous  InitialCondition=1  SampleTime=-1
  start : Outport
  end : Outport  Port=2
  valid : Outport  Port=3
  pop : Outport  Port=4
  advPop : Outport  Port=5
  wires:
  blockLen/1 -> Relational Operator/2, Add/1, Add1/1, Relational Operator2/2
  Delay/1 -> start/1, Unit Delay Enabled Synchronous/2, Unit Delay Enabled Synchronous1/2
  blockCount/1 -> Compare To Constant/1, Relational Operator/1, Relational Operator2/1, Relational Operator1/1, Relational Operator3/1
  Unit Delay Enabled Synchronous1/1 -> Logical Operator3/2
  Relational Operator3/1 -> Delay1/1
  Add1/1 -> Relational Operator3/2
  Constant2/1 -> Add1/2
  Constant3/1 -> Unit Delay Enabled Synchronous1/1
  Delay1/1 -> Logical Operator3/1
  Logical Operator3/1 -> advPop/1
  Unit Delay Enabled Synchronous/1 -> Logical Operator4/2
  Delay8/1 -> Logical Operator4/1
  Logical Operator4/1 -> pop/1
  Delay6/1 -> valid/1
  Delay5/1 -> end/1
  Constant1/1 -> Unit Delay Enabled Synchronous/1
  Compare To Constant/1 -> Logical Operator8/2
  Relational Operator1/1 -> Delay8/1
  Add/1 -> Relational Operator1/2
  Constant/1 -> Add/2
  Relational Operator2/1 -> Logical Operator1/2
  Relational Operator/1 -> Logical Operator2/2
  blockValid/1 -> Logical Operator8/1, Logical Operator2/1, Logical Operator1/1
  Logical Operator2/1 -> Delay5/1
  Logical Operator8/1 -> Delay/1
  Logical Operator1/1 -> Delay6/1

== system soc_WLAN_fpga/WLAN/WLAN HDL/WLAN_Tx_Rx/WLAN_Rx/WLANHDLReceiver/DataRecovery/Deinterleaver/DeInterleaver_NonHT/Stage 2 BPSK/Read Logic/Generate Read Address ==
  note: 1) Add Subsystem or Model blocks as valid variant choices.
      | 2) You cannot connect blocks at this level. At simulation, connectivity is automatically
      | determined, based on the active variant and port name matching.
  blockLen : Inport
  enable : Inport  Port=2
  reset : Inport  Port=3
  Read Address of Deinterleaver : Subsystem  VariantControl=isInterleaver==0
  Read Address of Interleaver : Subsystem  VariantControl=isInterleaver==1
  blockDataCount : Outport
  currentAddr : Outport  Port=2

== system soc_WLAN_fpga/WLAN/WLAN HDL/WLAN_Tx_Rx/WLAN_Rx/WLANHDLReceiver/DataRecovery/Deinterleaver/DeInterleaver_NonHT/Stage 2 BPSK/Write Logic/Generate Write Address ==
  rst : Inport
  enb : Inport  Port=2
  end : Inport  Port=3
  Add : Sum  OutDataTypeStr=Inherit: Inherit via back propagation
  Constant : Constant  Value=0  OutDataTypeStr=fixdt(0,nextpow2(maxBlkSize+1),0)  SampleTime=-1
  Constant4 : Constant  Value=maxBlkSize  OutDataTypeStr=fixdt(0,nextpow2(maxBlkSize+1),0)  SampleTime=-1
  HDL Counter : hdlsllib/Sources/HDL Counter  CountType=Count limited  CountInit=0  CountStep=1  CountMax=maxBlkSize  CountFromType=Initial value  CountFrom=0  CountResetPort=on  CountLoadPort=off  CountEnbPort=on  CountDirPort=off  CountHitOutputPort=off  CountDataType=Unsigned  CountWordLen=nextpow2(maxBlkSize+1)  CountFracLen=0  CountSampTime=1
  Logical Operator7 : Logic  Operator=NOT  IconShape=distinctive  AllPortsSameDT=off  OutDataTypeStr=boolean
  Switch : Switch  Criteria=u2 ~= 0  SaturateOnIntegerOverflow=off  InputSameDT=off
  Unit Delay Enabled Synchronous2 : hdlsllib/Discrete/Unit Delay Enabled Synchronous  InitialCondition=0  SampleTime=-1
  wrAddr : Outport
  count : Outport  Port=2
  wires:
  Logical Operator7/1 -> Unit Delay Enabled Synchronous2/1
  end/1 -> Unit Delay Enabled Synchronous2/2
  Unit Delay Enabled Synchronous2/1 -> Switch/2, Logical Operator7/1
  Add/1 -> wrAddr/1
  HDL Counter/1 -> count/1, Add/1  "currentAddr"
  rst/1 -> HDL Counter/1
  Constant/1 -> Switch/3
  Constant4/1 -> Switch/1
  enb/1 -> HDL Counter/2
  Switch/1 -> Add/2  "baseAddr"

== system soc_WLAN_fpga/WLAN/WLAN HDL/WLAN_Tx_Rx/WLAN_Rx/WLANHDLReceiver/DataRecovery/Deinterleaver/DeInterleaver_NonHT/Stage 2 BPSK/Write Logic/Handle Input Control Signals ==
  start : Inport
  valid : Inport  Port=2
  end : Inport  Port=3
  Delay{1..5} (5 alike) : Delay  DelayLength=1
  Generate Current Frame Status : Subsystem
  Generate Forced End : Subsystem
  Logical Operator : Logic  Operator=OR  IconShape=distinctive  AllPortsSameDT=off  OutDataTypeStr=boolean
  Logical Operator1 : Logic  Operator=NOT  IconShape=distinctive  AllPortsSameDT=off  OutDataTypeStr=boolean
  Logical Operator2 : Logic  IconShape=distinctive  AllPortsSameDT=off  OutDataTypeStr=boolean
  Logical Operator3 : Logic  Inputs=4  IconShape=distinctive  AllPortsSameDT=off  OutDataTypeStr=boolean
  Logical Operator5 : Logic  IconShape=distinctive  AllPortsSameDT=off  OutDataTypeStr=boolean
  reset : Outport
  countEnb : Outport  Port=2
  endOut : Outport  Port=3
  endReady : Outport  Port=4
  wires:
  Logical Operator1/1 -> Logical Operator3/4
  Logical Operator/1 -> Delay1/1, endReady/1
  Delay1/1 -> Generate Current Frame Status/2(end), Delay5/1, Logical Operator1/1
  Generate Forced End/1(forcedEnd) -> Logical Operator/2
  Logical Operator3/1 -> Logical Operator/1
  valid/1 -> Logical Operator3/1, Logical Operator2/2, Generate Forced End/2(valid), Delay4/1
  Delay5/1 -> endOut/1
  Delay3/1 -> countEnb/1
  Delay2/1 -> reset/1
  start/1 -> Logical Operator2/1
  Delay4/1 -> Logical Operator5/1
  end/1 -> Logical Operator3/2
  Logical Operator2/1 -> Generate Forced End/1(rst), Generate Current Frame Status/1(start), Delay2/1
  Generate Current Frame Status/1(frameOn) -> Generate Forced End/3(frameOn), Logical Operator3/3, Logical Operator5/2
  Logical Operator5/1 -> Delay3/1
